simulink model "motorPCtrl"  (R2016b)
settings: Solver=ode5  StartTime=0.0  StopTime=inf  FixedStep=0.001  RelTol=1e-3  EnableMultiTasking=on
undefined symbols (not defined in the file or in its folder): Humusoft, MF644
libraries: dcpctrl x2, sldrtlib x1
settings Model: SimulationMode=external  ExtModeArchiveFileName=dsaData  ExtModeArchiveDirName=/Users/julianleland/Documents/Git/GitHub/dcpctrl_v2/data/dsaData  ExtModeIncDirWhenArm=on  Creator=julianleland  LastModifiedBy=julianleland
settings DataIOCC: SaveOutput=off  SignalLogging=off  DSMLogging=off  SaveTime=off
settings OptimizationCC: LifeSpan=inf
settings DebuggingCC: SFUnexpectedBacktrackingDiag=warning  SFNoUnconditionalDefaultTransitionDiag=warning  SFExecutionAtInitializationDiag=none
settings HardwareCC: ProdBitPerLong=64  ProdHWDeviceType=Intel->x86-64 (Mac OS X)  TargetBitPerLong=64  TargetBitPerPointer=64  TargetIntDivRoundTo=Zero  TargetEndianess=LittleEndian  TargetWordSize=64  TargetHWDeviceType=Intel->x86-64
settings RTWCC: SystemTargetFile=sldrt.tlc  TemplateMakefile=sldrt.tmf  Description=Simulink Desktop Real-Time  RTWCompilerOptimization=on
settings CodeAppCC: MaxIdLength=95
settings SimulinkDesktopRealTimeCC: TargetPreCompLibLocation=/Applications/MATLAB_R2016b.app/toolbox/sldrt/lib/maci64  TargetLangStandard=C89/C90 (ANSI)  SupportVariableSizeSignals=off
settings ConfigComp: CovMetricSettings=dw  CovHtmlReporting=on  CovSaveCumulativeToWorkspaceVar=on  CovSaveSingleToWorkspaceVar=on  CovExternalEMLEnable=off

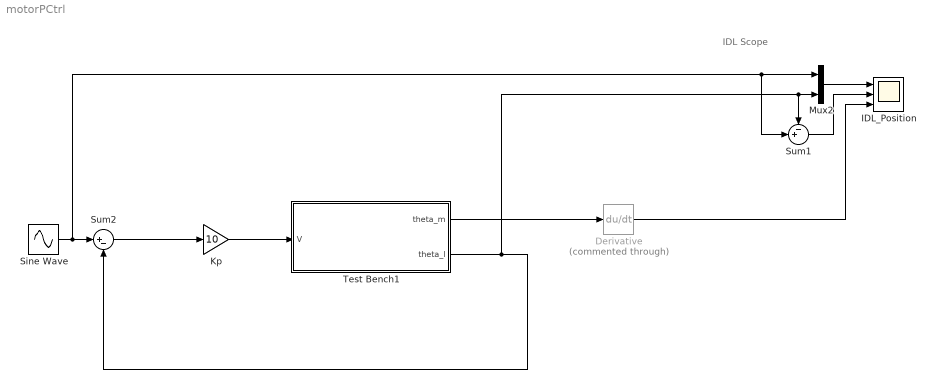
== system motorPCtrl ==
  note: IDL Scope
  Derivative : Derivative  Commented=through
  IDL_Position : Scope  NumInputPorts=3
  Kp : Gain  Gain=10
  Mux2 : Mux  Inputs=2
  Sine Wave : Sin  Amplitude=2  SampleTime=0
  Sum1 : Sum  Inputs=-+|
  Sum2 : Sum  Inputs=|+-
  Test Bench1 : Subsystem
  wires:
  Sum2/1 -> Kp/1
  Test Bench1/2(theta_l) -> Sum2/2, Sum1/1, Mux2/2
  Mux2/1 -> IDL_Position/1
  Sum1/1 -> IDL_Position/2
  Derivative/1 -> IDL_Position/3
  Sine Wave/1 -> Sum1/2, Mux2/1, Sum2/1
  Test Bench1/1(theta_m) -> Derivative/1
  Kp/1 -> Test Bench1/1(V)

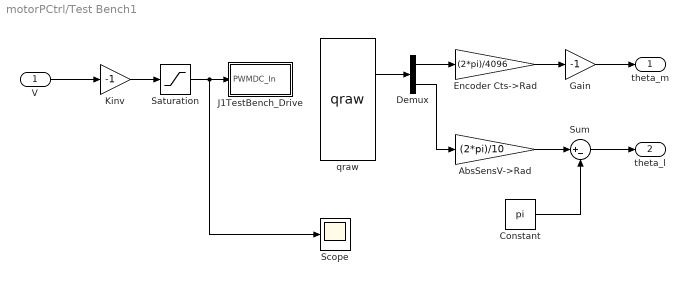
== system motorPCtrl/Test Bench1 ==
  V : Inport
  AbsSensV->Rad : Gain  Gain=(2*pi)/10
  Constant : Constant  Value=pi
  Demux : Demux  Outputs=2
  Encoder Cts->Rad : Gain  Gain=(2*pi)/4096
  Gain : Gain  Gain=-1
  J1TestBench_Drive : Subsystem
  Kinv : Gain  Gain=-1
  Saturation : Saturate  UpperLimit=1  LowerLimit=-1
  Scope : Scope
  Sum : Sum  Inputs=|+-
  qraw : dcpctrl/qraw
  theta_m : Outport
  theta_l : Outport  Port=2
  wires:
  Saturation/1 -> Scope/1, J1TestBench_Drive/1(PWMDC_In)
  Demux/1 -> Encoder Cts->Rad/1
  Kinv/1 -> Saturation/1
  Demux/2 -> AbsSensV->Rad/1
  V/1 -> Kinv/1
  qraw/2 -> Demux/1
  AbsSensV->Rad/1 -> Sum/1
  Sum/1 -> theta_l/1
  Constant/1 -> Sum/2
  Encoder Cts->Rad/1 -> Gain/1
  Gain/1 -> theta_m/1

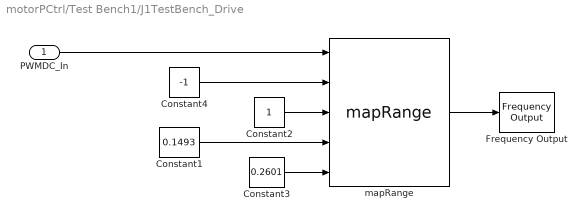
== system motorPCtrl/Test Bench1/J1TestBench_Drive ==
  PWMDC_In : Inport
  Constant1 : Constant  Value=0.1493
  Constant2 : Constant
  Constant3 : Constant  Value=0.2601
  Constant4 : Constant  Value=-1
  Frequency Output : sldrtlib/Frequency Output  SampleTime=-1  MaxMissedTicks=10  ShowMissedTicks=off  YieldWhenWaiting=off  DrvName=Humusoft/MF644  DrvAddress=4294967295  DrvOptions=585  Channels=1  FrequencySource=1  Frequency=150  FrequencyFinalValue=[]  DutySource=2  Duty=0.5  DutyFinalValue=0.5
      settings: AttributesFormatString=Humusoft\nMF644 [auto]
  "mapRange " : dcpctrl/mapRange 
  wires:
  Constant1/1 -> "mapRange "/4
  "mapRange "/1 -> Frequency Output/1
  PWMDC_In/1 -> "mapRange "/1
  Constant4/1 -> "mapRange "/2
  Constant3/1 -> "mapRange "/5
  Constant2/1 -> "mapRange "/3
